simulink model "firstorderresponse2"  (Simulink 7.4)
settings: Solver=ode45  StartTime=0.0  StopTime=3  RelTol=1e-3
settings Model: Creator=m136852  LastModifiedBy=m136852
settings DataIOCC: LimitDataPoints=off

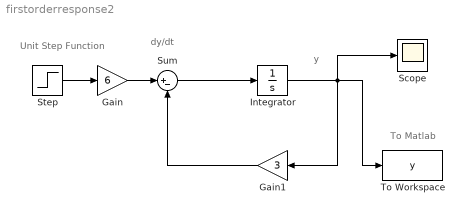
== system firstorderresponse2 ==
  note: To Matlab
  note: Unit Step Function
  note: dy/dt
  note: y
  Gain : Gain  Gain=6  ParameterDataType=fixdt(1, 16)  ParameterScaling=2^0  OutDataType=fixdt(1, 16)  OutScaling=2^0
  Gain1 : Gain  Gain=3  ParameterDataType=fixdt(1, 16)  ParameterScaling=2^0  OutDataType=fixdt(1, 16)  OutScaling=2^0
  Integrator : Integrator
  Scope : Scope
  Step : Step  Time=0  SampleTime=0
  Sum : Sum  Inputs=|+-  OutDataType=fixdt(1, 16)  OutScaling=2^0
  To Workspace : ToWorkspace  VariableName=y  SampleTime=-1  SaveFormat=Array
  wires:
  Step/1 -> Gain/1
  Gain1/1 -> Sum/2
  Gain/1 -> Sum/1
  Sum/1 -> Integrator/1
  Integrator/1 -> Gain1/1, Scope/1, To Workspace/1
